simulink model "Pokus07_Display"  (Simulink 8.1)
settings: Solver=ode45  StartTime=0.0  StopTime=10.0  RelTol=1e-3
undefined symbols (not defined in the file): A, ARROW_DOWN, ARROW_LEFT, ARROW_RIGHT, ARROW_UP, ASTERISK, B, BACKSLASH, C, COLON, COMMA, CROSS, CURSOR, D, DOT, ending_column_index, ending_row_index, EQUAL, EXCLAMATION_MARK, F, framebuffer, G, GREATER_THAN, H, HEIGHT, hot, I, J, K, L, LEFT_PARENTHESES, LESS_THAN, M, MINUS, N, O, P, PERCENT, PLUS, POS_X, POS_Y, Q, QUESTION_MARK, QUOTE, R, RECTANGLE, RIGHT_PARENTHESES, S, SEMICOLON, SHARP, SLASH, SPACE, starting_column_index, starting_row_index, T, U, UNDERSCORE, V, W, WIDTH ... (+6)
libraries: dspmtrx3 x197, Common_Library x69, commutil2 x53, simulink_extras x1, dspsnks4 x1
(part 2 of 6)

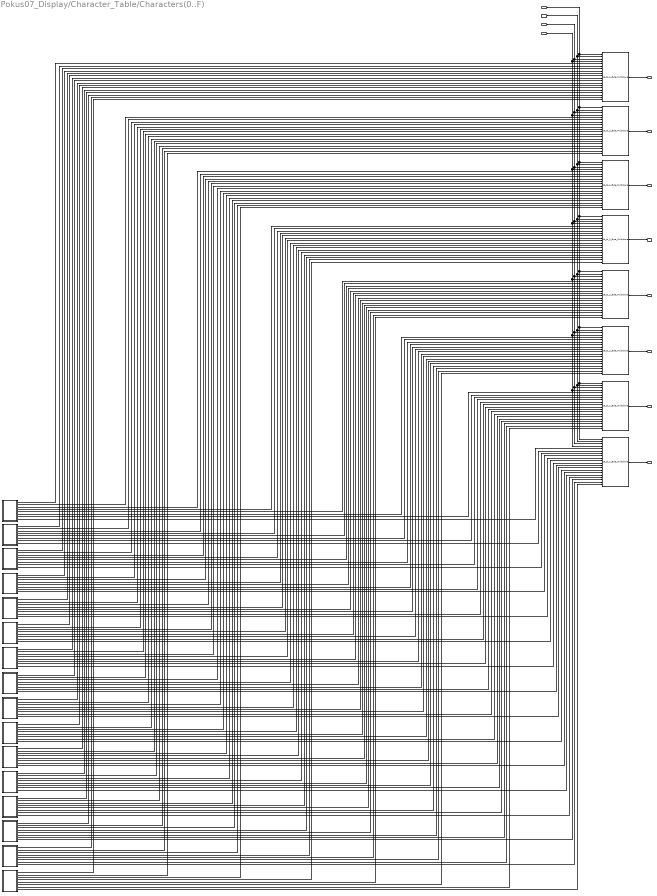
== system Pokus07_Display/Character_Table/Characters(0..F) ==
  Address_3_In(1b) : Inport
  Address_2_In(1b) : Inport  Port=2
  Address_1_In(1b) : Inport  Port=3
  Address_0_In(1b) : Inport  Port=4
  16_to_1_Byte_Multiplexer{,1..7} (8 alike) : Common_Library/Multiplexers/16_to_1_Byte_Multiplexer
  Char_0 : Subsystem
  Char_1 : Subsystem
  Char_2 : Subsystem
  Char_3 : Subsystem
  Char_4 : Subsystem
  Char_5 : Subsystem
  Char_6 : Subsystem
  Char_7 : Subsystem
  Char_8 : Subsystem
  Char_9 : Subsystem
  Char_A : Subsystem
  Char_B : Subsystem
  Char_C : Subsystem
  Char_D : Subsystem
  Char_E : Subsystem
  Char_F : Subsystem
  Column_1(1B) : Outport
  Column_2(1B) : Outport  Port=2
  Column_3(1B) : Outport  Port=3
  Column_4(1B) : Outport  Port=4
  Column_5(1B) : Outport  Port=5
  Column_6(1B) : Outport  Port=6
  Column_7(1B) : Outport  Port=7
  Column_8(1B) : Outport  Port=8
  wires:
  Char_F/1(Column_1(1B)) -> 16_to_1_Byte_Multiplexer/5
  Char_E/1(Column_1(1B)) -> 16_to_1_Byte_Multiplexer/6
  Char_D/1(Column_1(1B)) -> 16_to_1_Byte_Multiplexer/7
  Char_C/1(Column_1(1B)) -> 16_to_1_Byte_Multiplexer/8
  Char_B/1(Column_1(1B)) -> 16_to_1_Byte_Multiplexer/9
  Char_A/1(Column_1(1B)) -> 16_to_1_Byte_Multiplexer/10
  Char_9/1(Column_1(1B)) -> 16_to_1_Byte_Multiplexer/11
  Char_8/1(Column_1(1B)) -> 16_to_1_Byte_Multiplexer/12
  Char_7/1(Column_1(1B)) -> 16_to_1_Byte_Multiplexer/13
  Char_6/1(Column_1(1B)) -> 16_to_1_Byte_Multiplexer/14
  Char_5/1(Column_1(1B)) -> 16_to_1_Byte_Multiplexer/15
  Char_4/1(Column_1(1B)) -> 16_to_1_Byte_Multiplexer/16
  Char_3/1(Column_1(1B)) -> 16_to_1_Byte_Multiplexer/17
  Char_2/1(Column_1(1B)) -> 16_to_1_Byte_Multiplexer/18
  Char_1/1(Column_1(1B)) -> 16_to_1_Byte_Multiplexer/19
  Char_0/1(Column_1(1B)) -> 16_to_1_Byte_Multiplexer/20
  Char_F/2(Column_2(1B)) -> 16_to_1_Byte_Multiplexer1/5
  Char_0/2(Column_2(1B)) -> 16_to_1_Byte_Multiplexer1/20
  Char_1/2(Column_2(1B)) -> 16_to_1_Byte_Multiplexer1/19
  Char_2/2(Column_2(1B)) -> 16_to_1_Byte_Multiplexer1/18
  Char_3/2(Column_2(1B)) -> 16_to_1_Byte_Multiplexer1/17
  Char_4/2(Column_2(1B)) -> 16_to_1_Byte_Multiplexer1/16
  Char_5/2(Column_2(1B)) -> 16_to_1_Byte_Multiplexer1/15
  Char_6/2(Column_2(1B)) -> 16_to_1_Byte_Multiplexer1/14
  Char_7/2(Column_2(1B)) -> 16_to_1_Byte_Multiplexer1/13
  Char_8/2(Column_2(1B)) -> 16_to_1_Byte_Multiplexer1/12
  Char_9/2(Column_2(1B)) -> 16_to_1_Byte_Multiplexer1/11
  Char_A/2(Column_2(1B)) -> 16_to_1_Byte_Multiplexer1/10
  Char_B/2(Column_2(1B)) -> 16_to_1_Byte_Multiplexer1/9
  Char_C/2(Column_2(1B)) -> 16_to_1_Byte_Multiplexer1/8
  Char_D/2(Column_2(1B)) -> 16_to_1_Byte_Multiplexer1/7
  Char_E/2(Column_2(1B)) -> 16_to_1_Byte_Multiplexer1/6
  Char_0/3(Column_3(1B)) -> 16_to_1_Byte_Multiplexer2/20
  Char_1/3(Column_3(1B)) -> 16_to_1_Byte_Multiplexer2/19
  Char_2/3(Column_3(1B)) -> 16_to_1_Byte_Multiplexer2/18
  Char_3/3(Column_3(1B)) -> 16_to_1_Byte_Multiplexer2/17
  Char_4/3(Column_3(1B)) -> 16_to_1_Byte_Multiplexer2/16
  Char_5/3(Column_3(1B)) -> 16_to_1_Byte_Multiplexer2/15
  Char_6/3(Column_3(1B)) -> 16_to_1_Byte_Multiplexer2/14
  Char_7/3(Column_3(1B)) -> 16_to_1_Byte_Multiplexer2/13
  Char_8/3(Column_3(1B)) -> 16_to_1_Byte_Multiplexer2/12
  Char_9/3(Column_3(1B)) -> 16_to_1_Byte_Multiplexer2/11
  Char_A/3(Column_3(1B)) -> 16_to_1_Byte_Multiplexer2/10
  Char_B/3(Column_3(1B)) -> 16_to_1_Byte_Multiplexer2/9
  Char_C/3(Column_3(1B)) -> 16_to_1_Byte_Multiplexer2/8
  Char_D/3(Column_3(1B)) -> 16_to_1_Byte_Multiplexer2/7
  Char_E/3(Column_3(1B)) -> 16_to_1_Byte_Multiplexer2/6
  Char_F/3(Column_3(1B)) -> 16_to_1_Byte_Multiplexer2/5
  Char_0/4(Column_4(1B)) -> 16_to_1_Byte_Multiplexer3/20
  Char_1/4(Column_4(1B)) -> 16_to_1_Byte_Multiplexer3/19
  Char_2/4(Column_4(1B)) -> 16_to_1_Byte_Multiplexer3/18
  Char_3/4(Column_4(1B)) -> 16_to_1_Byte_Multiplexer3/17
  Char_4/4(Column_4(1B)) -> 16_to_1_Byte_Multiplexer3/16
  Char_5/4(Column_4(1B)) -> 16_to_1_Byte_Multiplexer3/15
  Char_6/4(Column_4(1B)) -> 16_to_1_Byte_Multiplexer3/14
  Char_7/4(Column_4(1B)) -> 16_to_1_Byte_Multiplexer3/13
  Char_8/4(Column_4(1B)) -> 16_to_1_Byte_Multiplexer3/12
  Char_9/4(Column_4(1B)) -> 16_to_1_Byte_Multiplexer3/11
  Char_A/4(Column_4(1B)) -> 16_to_1_Byte_Multiplexer3/10
  Char_B/4(Column_4(1B)) -> 16_to_1_Byte_Multiplexer3/9
  Char_C/4(Column_4(1B)) -> 16_to_1_Byte_Multiplexer3/8
  Char_D/4(Column_4(1B)) -> 16_to_1_Byte_Multiplexer3/7
  Char_E/4(Column_4(1B)) -> 16_to_1_Byte_Multiplexer3/6
  Char_F/4(Column_4(1B)) -> 16_to_1_Byte_Multiplexer3/5
  Char_0/5(Column_5(1B)) -> 16_to_1_Byte_Multiplexer4/20
  Char_1/5(Column_5(1B)) -> 16_to_1_Byte_Multiplexer4/19
  Char_2/5(Column_5(1B)) -> 16_to_1_Byte_Multiplexer4/18
  Char_3/5(Column_5(1B)) -> 16_to_1_Byte_Multiplexer4/17
  Char_4/5(Column_5(1B)) -> 16_to_1_Byte_Multiplexer4/16
  Char_5/5(Column_5(1B)) -> 16_to_1_Byte_Multiplexer4/15
  Char_7/5(Column_5(1B)) -> 16_to_1_Byte_Multiplexer4/13
  Char_6/5(Column_5(1B)) -> 16_to_1_Byte_Multiplexer4/14
  Char_8/5(Column_5(1B)) -> 16_to_1_Byte_Multiplexer4/12
  Char_9/5(Column_5(1B)) -> 16_to_1_Byte_Multiplexer4/11
  Char_A/5(Column_5(1B)) -> 16_to_1_Byte_Multiplexer4/10
  Char_B/5(Column_5(1B)) -> 16_to_1_Byte_Multiplexer4/9
  Char_C/5(Column_5(1B)) -> 16_to_1_Byte_Multiplexer4/8
  Char_D/5(Column_5(1B)) -> 16_to_1_Byte_Multiplexer4/7
  Char_E/5(Column_5(1B)) -> 16_to_1_Byte_Multiplexer4/6
  Char_F/5(Column_5(1B)) -> 16_to_1_Byte_Multiplexer4/5
  Char_0/6(Column_6(1B)) -> 16_to_1_Byte_Multiplexer5/20
  Char_1/6(Column_6(1B)) -> 16_to_1_Byte_Multiplexer5/19
  Char_2/6(Column_6(1B)) -> 16_to_1_Byte_Multiplexer5/18
  Char_3/6(Column_6(1B)) -> 16_to_1_Byte_Multiplexer5/17
  Char_4/6(Column_6(1B)) -> 16_to_1_Byte_Multiplexer5/16
  Char_5/6(Column_6(1B)) -> 16_to_1_Byte_Multiplexer5/15
  Char_6/6(Column_6(1B)) -> 16_to_1_Byte_Multiplexer5/14
  Char_7/6(Column_6(1B)) -> 16_to_1_Byte_Multiplexer5/13
  Char_8/6(Column_6(1B)) -> 16_to_1_Byte_Multiplexer5/12
  Char_9/6(Column_6(1B)) -> 16_to_1_Byte_Multiplexer5/11
  Char_A/6(Column_6(1B)) -> 16_to_1_Byte_Multiplexer5/10
  Char_B/6(Column_6(1B)) -> 16_to_1_Byte_Multiplexer5/9
  Char_C/7(Column_7(1B)) -> 16_to_1_Byte_Multiplexer6/8
  Char_C/6(Column_6(1B)) -> 16_to_1_Byte_Multiplexer5/8
  Char_D/6(Column_6(1B)) -> 16_to_1_Byte_Multiplexer5/7
  Char_E/6(Column_6(1B)) -> 16_to_1_Byte_Multiplexer5/6
  Char_F/6(Column_6(1B)) -> 16_to_1_Byte_Multiplexer5/5
  Char_0/7(Column_7(1B)) -> 16_to_1_Byte_Multiplexer6/20
  Char_1/7(Column_7(1B)) -> 16_to_1_Byte_Multiplexer6/19
  Char_2/7(Column_7(1B)) -> 16_to_1_Byte_Multiplexer6/18
  Char_3/7(Column_7(1B)) -> 16_to_1_Byte_Multiplexer6/17
  Char_4/7(Column_7(1B)) -> 16_to_1_Byte_Multiplexer6/16
  Char_5/7(Column_7(1B)) -> 16_to_1_Byte_Multiplexer6/15
  Char_6/7(Column_7(1B)) -> 16_to_1_Byte_Multiplexer6/14
  Char_7/7(Column_7(1B)) -> 16_to_1_Byte_Multiplexer6/13
  Char_8/7(Column_7(1B)) -> 16_to_1_Byte_Multiplexer6/12
  Char_9/7(Column_7(1B)) -> 16_to_1_Byte_Multiplexer6/11
  Char_A/7(Column_7(1B)) -> 16_to_1_Byte_Multiplexer6/10
  Char_B/7(Column_7(1B)) -> 16_to_1_Byte_Multiplexer6/9
  Char_D/7(Column_7(1B)) -> 16_to_1_Byte_Multiplexer6/7
  Char_E/7(Column_7(1B)) -> 16_to_1_Byte_Multiplexer6/6
  Char_F/7(Column_7(1B)) -> 16_to_1_Byte_Multiplexer6/5
  Char_0/8(Column_8(1B)) -> 16_to_1_Byte_Multiplexer7/20
  Char_1/8(Column_8(1B)) -> 16_to_1_Byte_Multiplexer7/19
  Char_2/8(Column_8(1B)) -> 16_to_1_Byte_Multiplexer7/18
  Char_3/8(Column_8(1B)) -> 16_to_1_Byte_Multiplexer7/17
  Char_4/8(Column_8(1B)) -> 16_to_1_Byte_Multiplexer7/16
  Char_5/8(Column_8(1B)) -> 16_to_1_Byte_Multiplexer7/15
  Char_6/8(Column_8(1B)) -> 16_to_1_Byte_Multiplexer7/14
  Char_7/8(Column_8(1B)) -> 16_to_1_Byte_Multiplexer7/13
  Char_8/8(Column_8(1B)) -> 16_to_1_Byte_Multiplexer7/12
  Char_9/8(Column_8(1B)) -> 16_to_1_Byte_Multiplexer7/11
  Char_A/8(Column_8(1B)) -> 16_to_1_Byte_Multiplexer7/10
  Char_B/8(Column_8(1B)) -> 16_to_1_Byte_Multiplexer7/9
  Char_C/8(Column_8(1B)) -> 16_to_1_Byte_Multiplexer7/8
  Char_D/8(Column_8(1B)) -> 16_to_1_Byte_Multiplexer7/7
  Char_E/8(Column_8(1B)) -> 16_to_1_Byte_Multiplexer7/6
  Char_F/8(Column_8(1B)) -> 16_to_1_Byte_Multiplexer7/5
  16_to_1_Byte_Multiplexer/1 -> Column_1(1B)/1
  16_to_1_Byte_Multiplexer1/1 -> Column_2(1B)/1
  16_to_1_Byte_Multiplexer2/1 -> Column_3(1B)/1
  16_to_1_Byte_Multiplexer3/1 -> Column_4(1B)/1
  16_to_1_Byte_Multiplexer4/1 -> Column_5(1B)/1
  16_to_1_Byte_Multiplexer5/1 -> Column_6(1B)/1
  16_to_1_Byte_Multiplexer6/1 -> Column_7(1B)/1
  16_to_1_Byte_Multiplexer7/1 -> Column_8(1B)/1
  Address_0_In(1b)/1 -> 16_to_1_Byte_Multiplexer/4, 16_to_1_Byte_Multiplexer1/4, 16_to_1_Byte_Multiplexer2/4, 16_to_1_Byte_Multiplexer3/4, 16_to_1_Byte_Multiplexer4/4, 16_to_1_Byte_Multiplexer5/4, 16_to_1_Byte_Multiplexer6/4, 16_to_1_Byte_Multiplexer7/4
  Address_1_In(1b)/1 -> 16_to_1_Byte_Multiplexer/3, 16_to_1_Byte_Multiplexer1/3, 16_to_1_Byte_Multiplexer2/3, 16_to_1_Byte_Multiplexer3/3, 16_to_1_Byte_Multiplexer4/3, 16_to_1_Byte_Multiplexer5/3, 16_to_1_Byte_Multiplexer6/3, 16_to_1_Byte_Multiplexer7/3
  Address_2_In(1b)/1 -> 16_to_1_Byte_Multiplexer/2, 16_to_1_Byte_Multiplexer1/2, 16_to_1_Byte_Multiplexer2/2, 16_to_1_Byte_Multiplexer3/2, 16_to_1_Byte_Multiplexer4/2, 16_to_1_Byte_Multiplexer5/2, 16_to_1_Byte_Multiplexer6/2, 16_to_1_Byte_Multiplexer7/2
  Address_3_In(1b)/1 -> 16_to_1_Byte_Multiplexer/1, 16_to_1_Byte_Multiplexer1/1, 16_to_1_Byte_Multiplexer2/1, 16_to_1_Byte_Multiplexer3/1, 16_to_1_Byte_Multiplexer4/1, 16_to_1_Byte_Multiplexer5/1, 16_to_1_Byte_Multiplexer6/1, 16_to_1_Byte_Multiplexer7/1

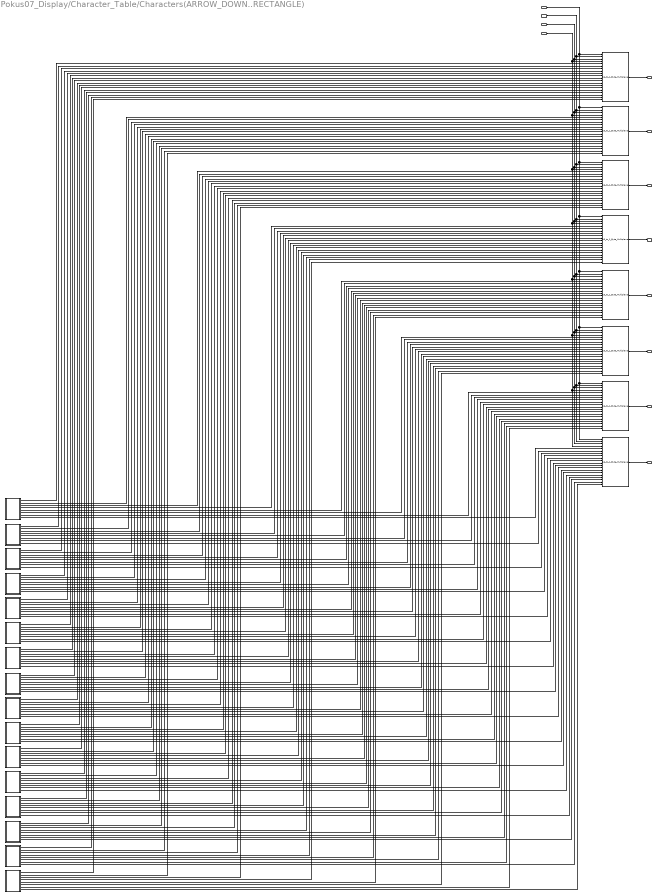
== system Pokus07_Display/Character_Table/Characters(ARROW_DOWN..RECTANGLE) ==
  Address_3_In(1b) : Inport
  Address_2_In(1b) : Inport  Port=2
  Address_1_In(1b) : Inport  Port=3
  Address_0_In(1b) : Inport  Port=4
  16_to_1_Byte_Multiplexer{,1..7} (8 alike) : Common_Library/Multiplexers/16_to_1_Byte_Multiplexer
  Char_ARROW_DOWN : Subsystem
  Char_ARROW_LEFT : Subsystem
  Char_ARROW_RIGHT : Subsystem
  Char_COMMA : Subsystem
  Char_CURSOR : Subsystem
  Char_DOT : Subsystem
  Char_EXCLAMATION_MARK : Subsystem
  Char_LEFT_PARENTHESES : Subsystem
  Char_PERCENT : Subsystem
  Char_QUESTION_MARK : Subsystem
  Char_QUOTE : Subsystem
  Char_RECTANGLE : Subsystem
  Char_RIGHT_PARENTHESES : Subsystem
  Char_SHARP : Subsystem
  Char_SPACE : Subsystem
  Char_UNDERSCORE : Subsystem
  Column_1(1B) : Outport
  Column_2(1B) : Outport  Port=2
  Column_3(1B) : Outport  Port=3
  Column_4(1B) : Outport  Port=4
  Column_5(1B) : Outport  Port=5
  Column_6(1B) : Outport  Port=6
  Column_7(1B) : Outport  Port=7
  Column_8(1B) : Outport  Port=8
  wires:
  Char_RECTANGLE/1(Column_1(1B)) -> 16_to_1_Byte_Multiplexer/5
  Char_CURSOR/1(Column_1(1B)) -> 16_to_1_Byte_Multiplexer/6
  Char_SPACE/1(Column_1(1B)) -> 16_to_1_Byte_Multiplexer/7
  Char_RIGHT_PARENTHESES/1(Column_1(1B)) -> 16_to_1_Byte_Multiplexer/8
  Char_LEFT_PARENTHESES/1(Column_1(1B)) -> 16_to_1_Byte_Multiplexer/9
  Char_PERCENT/1(Column_1(1B)) -> 16_to_1_Byte_Multiplexer/10
  Char_SHARP/1(Column_1(1B)) -> 16_to_1_Byte_Multiplexer/11
  Char_QUOTE/1(Column_1(1B)) -> 16_to_1_Byte_Multiplexer/12
  Char_EXCLAMATION_MARK/1(Column_1(1B)) -> 16_to_1_Byte_Multiplexer/13
  Char_QUESTION_MARK/1(Column_1(1B)) -> 16_to_1_Byte_Multiplexer/14
  Char_COMMA/1(Column_1(1B)) -> 16_to_1_Byte_Multiplexer/15
  Char_DOT/1(Column_1(1B)) -> 16_to_1_Byte_Multiplexer/16
  Char_UNDERSCORE/1(Column_1(1B)) -> 16_to_1_Byte_Multiplexer/17
  Char_ARROW_RIGHT/1(Column_1(1B)) -> 16_to_1_Byte_Multiplexer/18
  Char_ARROW_LEFT/1(Column_1(1B)) -> 16_to_1_Byte_Multiplexer/19
  Char_ARROW_DOWN/1(Column_1(1B)) -> 16_to_1_Byte_Multiplexer/20
  Char_RECTANGLE/2(Column_2(1B)) -> 16_to_1_Byte_Multiplexer1/5
  Char_ARROW_DOWN/2(Column_2(1B)) -> 16_to_1_Byte_Multiplexer1/20
  Char_ARROW_LEFT/2(Column_2(1B)) -> 16_to_1_Byte_Multiplexer1/19
  Char_ARROW_RIGHT/2(Column_2(1B)) -> 16_to_1_Byte_Multiplexer1/18
  Char_UNDERSCORE/2(Column_2(1B)) -> 16_to_1_Byte_Multiplexer1/17
  Char_DOT/2(Column_2(1B)) -> 16_to_1_Byte_Multiplexer1/16
  Char_COMMA/2(Column_2(1B)) -> 16_to_1_Byte_Multiplexer1/15
  Char_QUESTION_MARK/2(Column_2(1B)) -> 16_to_1_Byte_Multiplexer1/14
  Char_EXCLAMATION_MARK/2(Column_2(1B)) -> 16_to_1_Byte_Multiplexer1/13
  Char_QUOTE/2(Column_2(1B)) -> 16_to_1_Byte_Multiplexer1/12
  Char_SHARP/2(Column_2(1B)) -> 16_to_1_Byte_Multiplexer1/11
  Char_PERCENT/2(Column_2(1B)) -> 16_to_1_Byte_Multiplexer1/10
  Char_LEFT_PARENTHESES/2(Column_2(1B)) -> 16_to_1_Byte_Multiplexer1/9
  Char_RIGHT_PARENTHESES/2(Column_2(1B)) -> 16_to_1_Byte_Multiplexer1/8
  Char_SPACE/2(Column_2(1B)) -> 16_to_1_Byte_Multiplexer1/7
  Char_CURSOR/2(Column_2(1B)) -> 16_to_1_Byte_Multiplexer1/6
  Char_ARROW_DOWN/3(Column_3(1B)) -> 16_to_1_Byte_Multiplexer2/20
  Char_ARROW_LEFT/3(Column_3(1B)) -> 16_to_1_Byte_Multiplexer2/19
  Char_ARROW_RIGHT/3(Column_3(1B)) -> 16_to_1_Byte_Multiplexer2/18
  Char_UNDERSCORE/3(Column_3(1B)) -> 16_to_1_Byte_Multiplexer2/17
  Char_DOT/3(Column_3(1B)) -> 16_to_1_Byte_Multiplexer2/16
  Char_COMMA/3(Column_3(1B)) -> 16_to_1_Byte_Multiplexer2/15
  Char_QUESTION_MARK/3(Column_3(1B)) -> 16_to_1_Byte_Multiplexer2/14
  Char_EXCLAMATION_MARK/3(Column_3(1B)) -> 16_to_1_Byte_Multiplexer2/13
  Char_QUOTE/3(Column_3(1B)) -> 16_to_1_Byte_Multiplexer2/12
  Char_SHARP/3(Column_3(1B)) -> 16_to_1_Byte_Multiplexer2/11
  Char_PERCENT/3(Column_3(1B)) -> 16_to_1_Byte_Multiplexer2/10
  Char_LEFT_PARENTHESES/3(Column_3(1B)) -> 16_to_1_Byte_Multiplexer2/9
  Char_RIGHT_PARENTHESES/3(Column_3(1B)) -> 16_to_1_Byte_Multiplexer2/8
  Char_SPACE/3(Column_3(1B)) -> 16_to_1_Byte_Multiplexer2/7
  Char_CURSOR/3(Column_3(1B)) -> 16_to_1_Byte_Multiplexer2/6
  Char_RECTANGLE/3(Column_3(1B)) -> 16_to_1_Byte_Multiplexer2/5
  Char_ARROW_DOWN/4(Column_4(1B)) -> 16_to_1_Byte_Multiplexer3/20
  Char_ARROW_LEFT/4(Column_4(1B)) -> 16_to_1_Byte_Multiplexer3/19
  Char_ARROW_RIGHT/4(Column_4(1B)) -> 16_to_1_Byte_Multiplexer3/18
  Char_UNDERSCORE/4(Column_4(1B)) -> 16_to_1_Byte_Multiplexer3/17
  Char_DOT/4(Column_4(1B)) -> 16_to_1_Byte_Multiplexer3/16
  Char_COMMA/4(Column_4(1B)) -> 16_to_1_Byte_Multiplexer3/15
  Char_QUESTION_MARK/4(Column_4(1B)) -> 16_to_1_Byte_Multiplexer3/14
  Char_EXCLAMATION_MARK/4(Column_4(1B)) -> 16_to_1_Byte_Multiplexer3/13
  Char_QUOTE/4(Column_4(1B)) -> 16_to_1_Byte_Multiplexer3/12
  Char_SHARP/4(Column_4(1B)) -> 16_to_1_Byte_Multiplexer3/11
  Char_PERCENT/4(Column_4(1B)) -> 16_to_1_Byte_Multiplexer3/10
  Char_LEFT_PARENTHESES/4(Column_4(1B)) -> 16_to_1_Byte_Multiplexer3/9
  Char_RIGHT_PARENTHESES/4(Column_4(1B)) -> 16_to_1_Byte_Multiplexer3/8
  Char_SPACE/4(Column_4(1B)) -> 16_to_1_Byte_Multiplexer3/7
  Char_CURSOR/4(Column_4(1B)) -> 16_to_1_Byte_Multiplexer3/6
  Char_RECTANGLE/4(Column_4(1B)) -> 16_to_1_Byte_Multiplexer3/5
  Char_ARROW_DOWN/5(Column_5(1B)) -> 16_to_1_Byte_Multiplexer4/20
  Char_ARROW_LEFT/5(Column_5(1B)) -> 16_to_1_Byte_Multiplexer4/19
  Char_ARROW_RIGHT/5(Column_5(1B)) -> 16_to_1_Byte_Multiplexer4/18
  Char_UNDERSCORE/5(Column_5(1B)) -> 16_to_1_Byte_Multiplexer4/17
  Char_DOT/5(Column_5(1B)) -> 16_to_1_Byte_Multiplexer4/16
  Char_COMMA/5(Column_5(1B)) -> 16_to_1_Byte_Multiplexer4/15
  Char_EXCLAMATION_MARK/5(Column_5(1B)) -> 16_to_1_Byte_Multiplexer4/13
  Char_QUESTION_MARK/5(Column_5(1B)) -> 16_to_1_Byte_Multiplexer4/14
  Char_QUOTE/5(Column_5(1B)) -> 16_to_1_Byte_Multiplexer4/12
  Char_SHARP/5(Column_5(1B)) -> 16_to_1_Byte_Multiplexer4/11
  Char_PERCENT/5(Column_5(1B)) -> 16_to_1_Byte_Multiplexer4/10
  Char_LEFT_PARENTHESES/5(Column_5(1B)) -> 16_to_1_Byte_Multiplexer4/9
  Char_RIGHT_PARENTHESES/5(Column_5(1B)) -> 16_to_1_Byte_Multiplexer4/8
  Char_SPACE/5(Column_5(1B)) -> 16_to_1_Byte_Multiplexer4/7
  Char_CURSOR/5(Column_5(1B)) -> 16_to_1_Byte_Multiplexer4/6
  Char_RECTANGLE/5(Column_5(1B)) -> 16_to_1_Byte_Multiplexer4/5
  Char_ARROW_DOWN/6(Column_6(1B)) -> 16_to_1_Byte_Multiplexer5/20
  Char_ARROW_LEFT/6(Column_6(1B)) -> 16_to_1_Byte_Multiplexer5/19
  Char_ARROW_RIGHT/6(Column_6(1B)) -> 16_to_1_Byte_Multiplexer5/18
  Char_UNDERSCORE/6(Column_6(1B)) -> 16_to_1_Byte_Multiplexer5/17
  Char_DOT/6(Column_6(1B)) -> 16_to_1_Byte_Multiplexer5/16
  Char_COMMA/6(Column_6(1B)) -> 16_to_1_Byte_Multiplexer5/15
  Char_QUESTION_MARK/6(Column_6(1B)) -> 16_to_1_Byte_Multiplexer5/14
  Char_EXCLAMATION_MARK/6(Column_6(1B)) -> 16_to_1_Byte_Multiplexer5/13
  Char_QUOTE/6(Column_6(1B)) -> 16_to_1_Byte_Multiplexer5/12
  Char_SHARP/6(Column_6(1B)) -> 16_to_1_Byte_Multiplexer5/11
  Char_PERCENT/6(Column_6(1B)) -> 16_to_1_Byte_Multiplexer5/10
  Char_LEFT_PARENTHESES/6(Column_6(1B)) -> 16_to_1_Byte_Multiplexer5/9
  Char_RIGHT_PARENTHESES/7(Column_7(1B)) -> 16_to_1_Byte_Multiplexer6/8
  Char_RIGHT_PARENTHESES/6(Column_6(1B)) -> 16_to_1_Byte_Multiplexer5/8
  Char_SPACE/6(Column_6(1B)) -> 16_to_1_Byte_Multiplexer5/7
  Char_CURSOR/6(Column_6(1B)) -> 16_to_1_Byte_Multiplexer5/6
  Char_RECTANGLE/6(Column_6(1B)) -> 16_to_1_Byte_Multiplexer5/5
  Char_ARROW_DOWN/7(Column_7(1B)) -> 16_to_1_Byte_Multiplexer6/20
  Char_ARROW_LEFT/7(Column_7(1B)) -> 16_to_1_Byte_Multiplexer6/19
  Char_ARROW_RIGHT/7(Column_7(1B)) -> 16_to_1_Byte_Multiplexer6/18
  Char_UNDERSCORE/7(Column_7(1B)) -> 16_to_1_Byte_Multiplexer6/17
  Char_DOT/7(Column_7(1B)) -> 16_to_1_Byte_Multiplexer6/16
  Char_COMMA/7(Column_7(1B)) -> 16_to_1_Byte_Multiplexer6/15
  Char_QUESTION_MARK/7(Column_7(1B)) -> 16_to_1_Byte_Multiplexer6/14
  Char_EXCLAMATION_MARK/7(Column_7(1B)) -> 16_to_1_Byte_Multiplexer6/13
  Char_QUOTE/7(Column_7(1B)) -> 16_to_1_Byte_Multiplexer6/12
  Char_SHARP/7(Column_7(1B)) -> 16_to_1_Byte_Multiplexer6/11
  Char_PERCENT/7(Column_7(1B)) -> 16_to_1_Byte_Multiplexer6/10
  Char_LEFT_PARENTHESES/7(Column_7(1B)) -> 16_to_1_Byte_Multiplexer6/9
  Char_SPACE/7(Column_7(1B)) -> 16_to_1_Byte_Multiplexer6/7
  Char_CURSOR/7(Column_7(1B)) -> 16_to_1_Byte_Multiplexer6/6
  Char_RECTANGLE/7(Column_7(1B)) -> 16_to_1_Byte_Multiplexer6/5
  Char_ARROW_DOWN/8(Column_8(1B)) -> 16_to_1_Byte_Multiplexer7/20
  Char_ARROW_LEFT/8(Column_8(1B)) -> 16_to_1_Byte_Multiplexer7/19
  Char_ARROW_RIGHT/8(Column_8(1B)) -> 16_to_1_Byte_Multiplexer7/18
  Char_UNDERSCORE/8(Column_8(1B)) -> 16_to_1_Byte_Multiplexer7/17
  Char_DOT/8(Column_8(1B)) -> 16_to_1_Byte_Multiplexer7/16
  Char_COMMA/8(Column_8(1B)) -> 16_to_1_Byte_Multiplexer7/15
  Char_QUESTION_MARK/8(Column_8(1B)) -> 16_to_1_Byte_Multiplexer7/14
  Char_EXCLAMATION_MARK/8(Column_8(1B)) -> 16_to_1_Byte_Multiplexer7/13
  Char_QUOTE/8(Column_8(1B)) -> 16_to_1_Byte_Multiplexer7/12
  Char_SHARP/8(Column_8(1B)) -> 16_to_1_Byte_Multiplexer7/11
  Char_PERCENT/8(Column_8(1B)) -> 16_to_1_Byte_Multiplexer7/10
  Char_LEFT_PARENTHESES/8(Column_8(1B)) -> 16_to_1_Byte_Multiplexer7/9
  Char_RIGHT_PARENTHESES/8(Column_8(1B)) -> 16_to_1_Byte_Multiplexer7/8
  Char_SPACE/8(Column_8(1B)) -> 16_to_1_Byte_Multiplexer7/7
  Char_CURSOR/8(Column_8(1B)) -> 16_to_1_Byte_Multiplexer7/6
  Char_RECTANGLE/8(Column_8(1B)) -> 16_to_1_Byte_Multiplexer7/5
  16_to_1_Byte_Multiplexer/1 -> Column_1(1B)/1
  16_to_1_Byte_Multiplexer1/1 -> Column_2(1B)/1
  16_to_1_Byte_Multiplexer2/1 -> Column_3(1B)/1
  16_to_1_Byte_Multiplexer3/1 -> Column_4(1B)/1
  16_to_1_Byte_Multiplexer4/1 -> Column_5(1B)/1
  16_to_1_Byte_Multiplexer5/1 -> Column_6(1B)/1
  16_to_1_Byte_Multiplexer6/1 -> Column_7(1B)/1
  16_to_1_Byte_Multiplexer7/1 -> Column_8(1B)/1
  Address_0_In(1b)/1 -> 16_to_1_Byte_Multiplexer/4, 16_to_1_Byte_Multiplexer1/4, 16_to_1_Byte_Multiplexer2/4, 16_to_1_Byte_Multiplexer3/4, 16_to_1_Byte_Multiplexer4/4, 16_to_1_Byte_Multiplexer5/4, 16_to_1_Byte_Multiplexer6/4, 16_to_1_Byte_Multiplexer7/4
  Address_1_In(1b)/1 -> 16_to_1_Byte_Multiplexer/3, 16_to_1_Byte_Multiplexer1/3, 16_to_1_Byte_Multiplexer2/3, 16_to_1_Byte_Multiplexer3/3, 16_to_1_Byte_Multiplexer4/3, 16_to_1_Byte_Multiplexer5/3, 16_to_1_Byte_Multiplexer6/3, 16_to_1_Byte_Multiplexer7/3
  Address_2_In(1b)/1 -> 16_to_1_Byte_Multiplexer/2, 16_to_1_Byte_Multiplexer1/2, 16_to_1_Byte_Multiplexer2/2, 16_to_1_Byte_Multiplexer3/2, 16_to_1_Byte_Multiplexer4/2, 16_to_1_Byte_Multiplexer5/2, 16_to_1_Byte_Multiplexer6/2, 16_to_1_Byte_Multiplexer7/2
  Address_3_In(1b)/1 -> 16_to_1_Byte_Multiplexer/1, 16_to_1_Byte_Multiplexer1/1, 16_to_1_Byte_Multiplexer2/1, 16_to_1_Byte_Multiplexer3/1, 16_to_1_Byte_Multiplexer4/1, 16_to_1_Byte_Multiplexer5/1, 16_to_1_Byte_Multiplexer6/1, 16_to_1_Byte_Multiplexer7/1

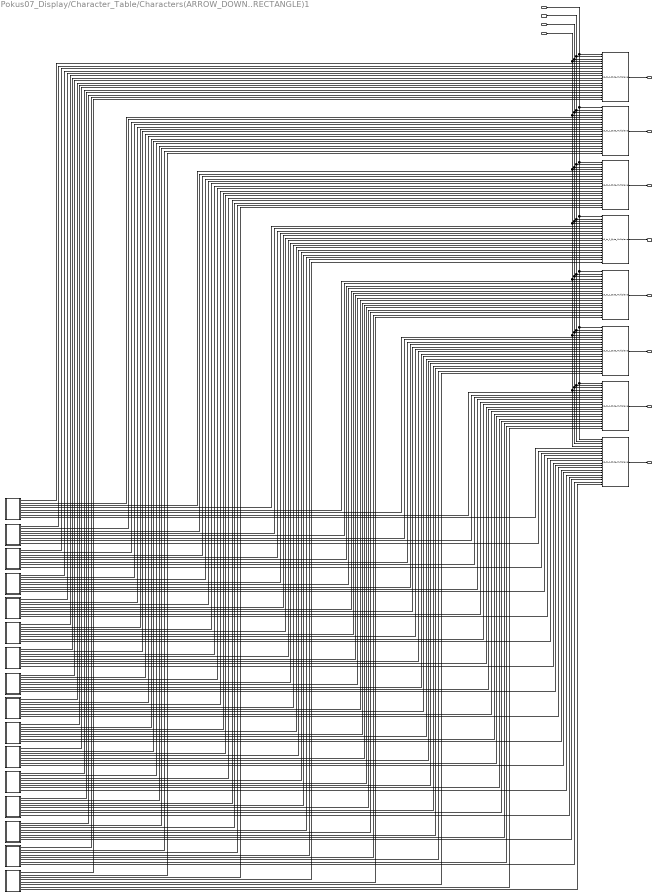
== system Pokus07_Display/Character_Table/Characters(ARROW_DOWN..RECTANGLE)1 ==
  Address_3_In(1b) : Inport
  Address_2_In(1b) : Inport  Port=2
  Address_1_In(1b) : Inport  Port=3
  Address_0_In(1b) : Inport  Port=4
  16_to_1_Byte_Multiplexer{,1..7} (8 alike) : Common_Library/Multiplexers/16_to_1_Byte_Multiplexer
  Char_ARROW_DOWN : Subsystem
  Char_ARROW_LEFT : Subsystem
  Char_ARROW_RIGHT : Subsystem
  Char_COMMA : Subsystem
  Char_CURSOR : Subsystem
  Char_DOT : Subsystem
  Char_EXCLAMATION_MARK : Subsystem
  Char_LEFT_PARENTHESES : Subsystem
  Char_PERCENT : Subsystem
  Char_QUESTION_MARK : Subsystem
  Char_QUOTE : Subsystem
  Char_RECTANGLE : Subsystem
  Char_RIGHT_PARENTHESES : Subsystem
  Char_SHARP : Subsystem
  Char_SPACE : Subsystem
  Char_UNDERSCORE : Subsystem
  Column_1(1B) : Outport
  Column_2(1B) : Outport  Port=2
  Column_3(1B) : Outport  Port=3
  Column_4(1B) : Outport  Port=4
  Column_5(1B) : Outport  Port=5
  Column_6(1B) : Outport  Port=6
  Column_7(1B) : Outport  Port=7
  Column_8(1B) : Outport  Port=8
  wires:
  Char_RECTANGLE/1(Column_1(1B)) -> 16_to_1_Byte_Multiplexer/5
  Char_CURSOR/1(Column_1(1B)) -> 16_to_1_Byte_Multiplexer/6
  Char_SPACE/1(Column_1(1B)) -> 16_to_1_Byte_Multiplexer/7
  Char_RIGHT_PARENTHESES/1(Column_1(1B)) -> 16_to_1_Byte_Multiplexer/8
  Char_LEFT_PARENTHESES/1(Column_1(1B)) -> 16_to_1_Byte_Multiplexer/9
  Char_PERCENT/1(Column_1(1B)) -> 16_to_1_Byte_Multiplexer/10
  Char_SHARP/1(Column_1(1B)) -> 16_to_1_Byte_Multiplexer/11
  Char_QUOTE/1(Column_1(1B)) -> 16_to_1_Byte_Multiplexer/12
  Char_EXCLAMATION_MARK/1(Column_1(1B)) -> 16_to_1_Byte_Multiplexer/13
  Char_QUESTION_MARK/1(Column_1(1B)) -> 16_to_1_Byte_Multiplexer/14
  Char_COMMA/1(Column_1(1B)) -> 16_to_1_Byte_Multiplexer/15
  Char_DOT/1(Column_1(1B)) -> 16_to_1_Byte_Multiplexer/16
  Char_UNDERSCORE/1(Column_1(1B)) -> 16_to_1_Byte_Multiplexer/17
  Char_ARROW_RIGHT/1(Column_1(1B)) -> 16_to_1_Byte_Multiplexer/18
  Char_ARROW_LEFT/1(Column_1(1B)) -> 16_to_1_Byte_Multiplexer/19
  Char_ARROW_DOWN/1(Column_1(1B)) -> 16_to_1_Byte_Multiplexer/20
  Char_RECTANGLE/2(Column_2(1B)) -> 16_to_1_Byte_Multiplexer1/5
  Char_ARROW_DOWN/2(Column_2(1B)) -> 16_to_1_Byte_Multiplexer1/20
  Char_ARROW_LEFT/2(Column_2(1B)) -> 16_to_1_Byte_Multiplexer1/19
  Char_ARROW_RIGHT/2(Column_2(1B)) -> 16_to_1_Byte_Multiplexer1/18
  Char_UNDERSCORE/2(Column_2(1B)) -> 16_to_1_Byte_Multiplexer1/17
  Char_DOT/2(Column_2(1B)) -> 16_to_1_Byte_Multiplexer1/16
  Char_COMMA/2(Column_2(1B)) -> 16_to_1_Byte_Multiplexer1/15
  Char_QUESTION_MARK/2(Column_2(1B)) -> 16_to_1_Byte_Multiplexer1/14
  Char_EXCLAMATION_MARK/2(Column_2(1B)) -> 16_to_1_Byte_Multiplexer1/13
  Char_QUOTE/2(Column_2(1B)) -> 16_to_1_Byte_Multiplexer1/12
  Char_SHARP/2(Column_2(1B)) -> 16_to_1_Byte_Multiplexer1/11
  Char_PERCENT/2(Column_2(1B)) -> 16_to_1_Byte_Multiplexer1/10
  Char_LEFT_PARENTHESES/2(Column_2(1B)) -> 16_to_1_Byte_Multiplexer1/9
  Char_RIGHT_PARENTHESES/2(Column_2(1B)) -> 16_to_1_Byte_Multiplexer1/8
  Char_SPACE/2(Column_2(1B)) -> 16_to_1_Byte_Multiplexer1/7
  Char_CURSOR/2(Column_2(1B)) -> 16_to_1_Byte_Multiplexer1/6
  Char_ARROW_DOWN/3(Column_3(1B)) -> 16_to_1_Byte_Multiplexer2/20
  Char_ARROW_LEFT/3(Column_3(1B)) -> 16_to_1_Byte_Multiplexer2/19
  Char_ARROW_RIGHT/3(Column_3(1B)) -> 16_to_1_Byte_Multiplexer2/18
  Char_UNDERSCORE/3(Column_3(1B)) -> 16_to_1_Byte_Multiplexer2/17
  Char_DOT/3(Column_3(1B)) -> 16_to_1_Byte_Multiplexer2/16
  Char_COMMA/3(Column_3(1B)) -> 16_to_1_Byte_Multiplexer2/15
  Char_QUESTION_MARK/3(Column_3(1B)) -> 16_to_1_Byte_Multiplexer2/14
  Char_EXCLAMATION_MARK/3(Column_3(1B)) -> 16_to_1_Byte_Multiplexer2/13
  Char_QUOTE/3(Column_3(1B)) -> 16_to_1_Byte_Multiplexer2/12
  Char_SHARP/3(Column_3(1B)) -> 16_to_1_Byte_Multiplexer2/11
  Char_PERCENT/3(Column_3(1B)) -> 16_to_1_Byte_Multiplexer2/10
  Char_LEFT_PARENTHESES/3(Column_3(1B)) -> 16_to_1_Byte_Multiplexer2/9
  Char_RIGHT_PARENTHESES/3(Column_3(1B)) -> 16_to_1_Byte_Multiplexer2/8
  Char_SPACE/3(Column_3(1B)) -> 16_to_1_Byte_Multiplexer2/7
  Char_CURSOR/3(Column_3(1B)) -> 16_to_1_Byte_Multiplexer2/6
  Char_RECTANGLE/3(Column_3(1B)) -> 16_to_1_Byte_Multiplexer2/5
  Char_ARROW_DOWN/4(Column_4(1B)) -> 16_to_1_Byte_Multiplexer3/20
  Char_ARROW_LEFT/4(Column_4(1B)) -> 16_to_1_Byte_Multiplexer3/19
  Char_ARROW_RIGHT/4(Column_4(1B)) -> 16_to_1_Byte_Multiplexer3/18
  Char_UNDERSCORE/4(Column_4(1B)) -> 16_to_1_Byte_Multiplexer3/17
  Char_DOT/4(Column_4(1B)) -> 16_to_1_Byte_Multiplexer3/16
  Char_COMMA/4(Column_4(1B)) -> 16_to_1_Byte_Multiplexer3/15
  Char_QUESTION_MARK/4(Column_4(1B)) -> 16_to_1_Byte_Multiplexer3/14
  Char_EXCLAMATION_MARK/4(Column_4(1B)) -> 16_to_1_Byte_Multiplexer3/13
  Char_QUOTE/4(Column_4(1B)) -> 16_to_1_Byte_Multiplexer3/12
  Char_SHARP/4(Column_4(1B)) -> 16_to_1_Byte_Multiplexer3/11
  Char_PERCENT/4(Column_4(1B)) -> 16_to_1_Byte_Multiplexer3/10
  Char_LEFT_PARENTHESES/4(Column_4(1B)) -> 16_to_1_Byte_Multiplexer3/9
  Char_RIGHT_PARENTHESES/4(Column_4(1B)) -> 16_to_1_Byte_Multiplexer3/8
  Char_SPACE/4(Column_4(1B)) -> 16_to_1_Byte_Multiplexer3/7
  Char_CURSOR/4(Column_4(1B)) -> 16_to_1_Byte_Multiplexer3/6
  Char_RECTANGLE/4(Column_4(1B)) -> 16_to_1_Byte_Multiplexer3/5
  Char_ARROW_DOWN/5(Column_5(1B)) -> 16_to_1_Byte_Multiplexer4/20
  Char_ARROW_LEFT/5(Column_5(1B)) -> 16_to_1_Byte_Multiplexer4/19
  Char_ARROW_RIGHT/5(Column_5(1B)) -> 16_to_1_Byte_Multiplexer4/18
  Char_UNDERSCORE/5(Column_5(1B)) -> 16_to_1_Byte_Multiplexer4/17
  Char_DOT/5(Column_5(1B)) -> 16_to_1_Byte_Multiplexer4/16
  Char_COMMA/5(Column_5(1B)) -> 16_to_1_Byte_Multiplexer4/15
  Char_EXCLAMATION_MARK/5(Column_5(1B)) -> 16_to_1_Byte_Multiplexer4/13
  Char_QUESTION_MARK/5(Column_5(1B)) -> 16_to_1_Byte_Multiplexer4/14
  Char_QUOTE/5(Column_5(1B)) -> 16_to_1_Byte_Multiplexer4/12
  Char_SHARP/5(Column_5(1B)) -> 16_to_1_Byte_Multiplexer4/11
  Char_PERCENT/5(Column_5(1B)) -> 16_to_1_Byte_Multiplexer4/10
  Char_LEFT_PARENTHESES/5(Column_5(1B)) -> 16_to_1_Byte_Multiplexer4/9
  Char_RIGHT_PARENTHESES/5(Column_5(1B)) -> 16_to_1_Byte_Multiplexer4/8
  Char_SPACE/5(Column_5(1B)) -> 16_to_1_Byte_Multiplexer4/7
  Char_CURSOR/5(Column_5(1B)) -> 16_to_1_Byte_Multiplexer4/6
  Char_RECTANGLE/5(Column_5(1B)) -> 16_to_1_Byte_Multiplexer4/5
  Char_ARROW_DOWN/6(Column_6(1B)) -> 16_to_1_Byte_Multiplexer5/20
  Char_ARROW_LEFT/6(Column_6(1B)) -> 16_to_1_Byte_Multiplexer5/19
  Char_ARROW_RIGHT/6(Column_6(1B)) -> 16_to_1_Byte_Multiplexer5/18
  Char_UNDERSCORE/6(Column_6(1B)) -> 16_to_1_Byte_Multiplexer5/17
  Char_DOT/6(Column_6(1B)) -> 16_to_1_Byte_Multiplexer5/16
  Char_COMMA/6(Column_6(1B)) -> 16_to_1_Byte_Multiplexer5/15
  Char_QUESTION_MARK/6(Column_6(1B)) -> 16_to_1_Byte_Multiplexer5/14
  Char_EXCLAMATION_MARK/6(Column_6(1B)) -> 16_to_1_Byte_Multiplexer5/13
  Char_QUOTE/6(Column_6(1B)) -> 16_to_1_Byte_Multiplexer5/12
  Char_SHARP/6(Column_6(1B)) -> 16_to_1_Byte_Multiplexer5/11
  Char_PERCENT/6(Column_6(1B)) -> 16_to_1_Byte_Multiplexer5/10
  Char_LEFT_PARENTHESES/6(Column_6(1B)) -> 16_to_1_Byte_Multiplexer5/9
  Char_RIGHT_PARENTHESES/7(Column_7(1B)) -> 16_to_1_Byte_Multiplexer6/8
  Char_RIGHT_PARENTHESES/6(Column_6(1B)) -> 16_to_1_Byte_Multiplexer5/8
  Char_SPACE/6(Column_6(1B)) -> 16_to_1_Byte_Multiplexer5/7
  Char_CURSOR/6(Column_6(1B)) -> 16_to_1_Byte_Multiplexer5/6
  Char_RECTANGLE/6(Column_6(1B)) -> 16_to_1_Byte_Multiplexer5/5
  Char_ARROW_DOWN/7(Column_7(1B)) -> 16_to_1_Byte_Multiplexer6/20
  Char_ARROW_LEFT/7(Column_7(1B)) -> 16_to_1_Byte_Multiplexer6/19
  Char_ARROW_RIGHT/7(Column_7(1B)) -> 16_to_1_Byte_Multiplexer6/18
  Char_UNDERSCORE/7(Column_7(1B)) -> 16_to_1_Byte_Multiplexer6/17
  Char_DOT/7(Column_7(1B)) -> 16_to_1_Byte_Multiplexer6/16
  Char_COMMA/7(Column_7(1B)) -> 16_to_1_Byte_Multiplexer6/15
  Char_QUESTION_MARK/7(Column_7(1B)) -> 16_to_1_Byte_Multiplexer6/14
  Char_EXCLAMATION_MARK/7(Column_7(1B)) -> 16_to_1_Byte_Multiplexer6/13
  Char_QUOTE/7(Column_7(1B)) -> 16_to_1_Byte_Multiplexer6/12
  Char_SHARP/7(Column_7(1B)) -> 16_to_1_Byte_Multiplexer6/11
  Char_PERCENT/7(Column_7(1B)) -> 16_to_1_Byte_Multiplexer6/10
  Char_LEFT_PARENTHESES/7(Column_7(1B)) -> 16_to_1_Byte_Multiplexer6/9
  Char_SPACE/7(Column_7(1B)) -> 16_to_1_Byte_Multiplexer6/7
  Char_CURSOR/7(Column_7(1B)) -> 16_to_1_Byte_Multiplexer6/6
  Char_RECTANGLE/7(Column_7(1B)) -> 16_to_1_Byte_Multiplexer6/5
  Char_ARROW_DOWN/8(Column_8(1B)) -> 16_to_1_Byte_Multiplexer7/20
  Char_ARROW_LEFT/8(Column_8(1B)) -> 16_to_1_Byte_Multiplexer7/19
  Char_ARROW_RIGHT/8(Column_8(1B)) -> 16_to_1_Byte_Multiplexer7/18
  Char_UNDERSCORE/8(Column_8(1B)) -> 16_to_1_Byte_Multiplexer7/17
  Char_DOT/8(Column_8(1B)) -> 16_to_1_Byte_Multiplexer7/16
  Char_COMMA/8(Column_8(1B)) -> 16_to_1_Byte_Multiplexer7/15
  Char_QUESTION_MARK/8(Column_8(1B)) -> 16_to_1_Byte_Multiplexer7/14
  Char_EXCLAMATION_MARK/8(Column_8(1B)) -> 16_to_1_Byte_Multiplexer7/13
  Char_QUOTE/8(Column_8(1B)) -> 16_to_1_Byte_Multiplexer7/12
  Char_SHARP/8(Column_8(1B)) -> 16_to_1_Byte_Multiplexer7/11
  Char_PERCENT/8(Column_8(1B)) -> 16_to_1_Byte_Multiplexer7/10
  Char_LEFT_PARENTHESES/8(Column_8(1B)) -> 16_to_1_Byte_Multiplexer7/9
  Char_RIGHT_PARENTHESES/8(Column_8(1B)) -> 16_to_1_Byte_Multiplexer7/8
  Char_SPACE/8(Column_8(1B)) -> 16_to_1_Byte_Multiplexer7/7
  Char_CURSOR/8(Column_8(1B)) -> 16_to_1_Byte_Multiplexer7/6
  Char_RECTANGLE/8(Column_8(1B)) -> 16_to_1_Byte_Multiplexer7/5
  16_to_1_Byte_Multiplexer/1 -> Column_1(1B)/1
  16_to_1_Byte_Multiplexer1/1 -> Column_2(1B)/1
  16_to_1_Byte_Multiplexer2/1 -> Column_3(1B)/1
  16_to_1_Byte_Multiplexer3/1 -> Column_4(1B)/1
  16_to_1_Byte_Multiplexer4/1 -> Column_5(1B)/1
  16_to_1_Byte_Multiplexer5/1 -> Column_6(1B)/1
  16_to_1_Byte_Multiplexer6/1 -> Column_7(1B)/1
  16_to_1_Byte_Multiplexer7/1 -> Column_8(1B)/1
  Address_0_In(1b)/1 -> 16_to_1_Byte_Multiplexer/4, 16_to_1_Byte_Multiplexer1/4, 16_to_1_Byte_Multiplexer2/4, 16_to_1_Byte_Multiplexer3/4, 16_to_1_Byte_Multiplexer4/4, 16_to_1_Byte_Multiplexer5/4, 16_to_1_Byte_Multiplexer6/4, 16_to_1_Byte_Multiplexer7/4
  Address_1_In(1b)/1 -> 16_to_1_Byte_Multiplexer/3, 16_to_1_Byte_Multiplexer1/3, 16_to_1_Byte_Multiplexer2/3, 16_to_1_Byte_Multiplexer3/3, 16_to_1_Byte_Multiplexer4/3, 16_to_1_Byte_Multiplexer5/3, 16_to_1_Byte_Multiplexer6/3, 16_to_1_Byte_Multiplexer7/3
  Address_2_In(1b)/1 -> 16_to_1_Byte_Multiplexer/2, 16_to_1_Byte_Multiplexer1/2, 16_to_1_Byte_Multiplexer2/2, 16_to_1_Byte_Multiplexer3/2, 16_to_1_Byte_Multiplexer4/2, 16_to_1_Byte_Multiplexer5/2, 16_to_1_Byte_Multiplexer6/2, 16_to_1_Byte_Multiplexer7/2
  Address_3_In(1b)/1 -> 16_to_1_Byte_Multiplexer/1, 16_to_1_Byte_Multiplexer1/1, 16_to_1_Byte_Multiplexer2/1, 16_to_1_Byte_Multiplexer3/1, 16_to_1_Byte_Multiplexer4/1, 16_to_1_Byte_Multiplexer5/1, 16_to_1_Byte_Multiplexer6/1, 16_to_1_Byte_Multiplexer7/1

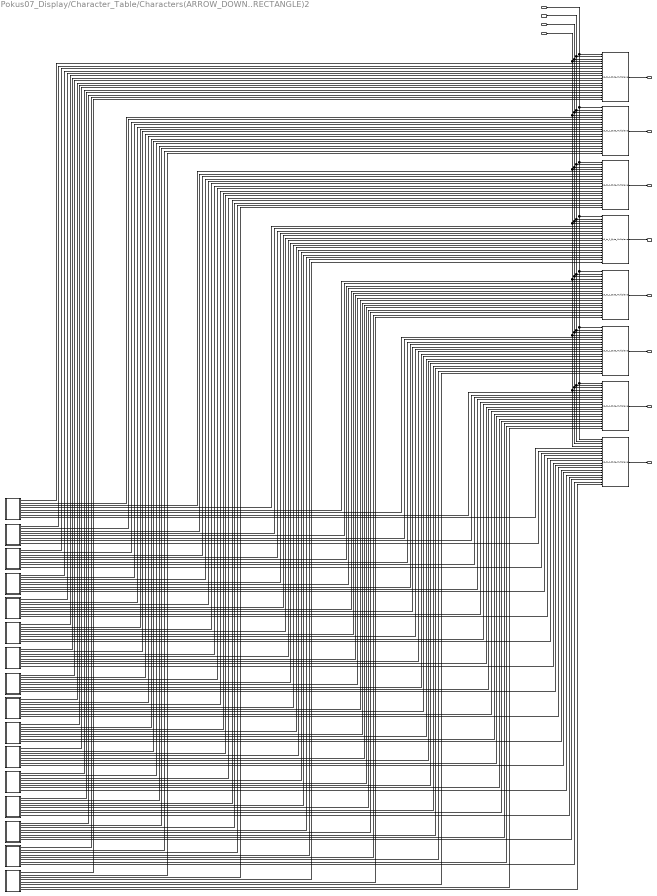
== system Pokus07_Display/Character_Table/Characters(ARROW_DOWN..RECTANGLE)2 ==
  Address_3_In(1b) : Inport
  Address_2_In(1b) : Inport  Port=2
  Address_1_In(1b) : Inport  Port=3
  Address_0_In(1b) : Inport  Port=4
  16_to_1_Byte_Multiplexer{,1..7} (8 alike) : Common_Library/Multiplexers/16_to_1_Byte_Multiplexer
  Char_ARROW_DOWN : Subsystem
  Char_ARROW_LEFT : Subsystem
  Char_ARROW_RIGHT : Subsystem
  Char_COMMA : Subsystem
  Char_CURSOR : Subsystem
  Char_DOT : Subsystem
  Char_EXCLAMATION_MARK : Subsystem
  Char_LEFT_PARENTHESES : Subsystem
  Char_PERCENT : Subsystem
  Char_QUESTION_MARK : Subsystem
  Char_QUOTE : Subsystem
  Char_RECTANGLE : Subsystem
  Char_RIGHT_PARENTHESES : Subsystem
  Char_SHARP : Subsystem
  Char_SPACE : Subsystem
  Char_UNDERSCORE : Subsystem
  Column_1(1B) : Outport
  Column_2(1B) : Outport  Port=2
  Column_3(1B) : Outport  Port=3
  Column_4(1B) : Outport  Port=4
  Column_5(1B) : Outport  Port=5
  Column_6(1B) : Outport  Port=6
  Column_7(1B) : Outport  Port=7
  Column_8(1B) : Outport  Port=8
  wires:
  Char_RECTANGLE/1(Column_1(1B)) -> 16_to_1_Byte_Multiplexer/5
  Char_CURSOR/1(Column_1(1B)) -> 16_to_1_Byte_Multiplexer/6
  Char_SPACE/1(Column_1(1B)) -> 16_to_1_Byte_Multiplexer/7
  Char_RIGHT_PARENTHESES/1(Column_1(1B)) -> 16_to_1_Byte_Multiplexer/8
  Char_LEFT_PARENTHESES/1(Column_1(1B)) -> 16_to_1_Byte_Multiplexer/9
  Char_PERCENT/1(Column_1(1B)) -> 16_to_1_Byte_Multiplexer/10
  Char_SHARP/1(Column_1(1B)) -> 16_to_1_Byte_Multiplexer/11
  Char_QUOTE/1(Column_1(1B)) -> 16_to_1_Byte_Multiplexer/12
  Char_EXCLAMATION_MARK/1(Column_1(1B)) -> 16_to_1_Byte_Multiplexer/13
  Char_QUESTION_MARK/1(Column_1(1B)) -> 16_to_1_Byte_Multiplexer/14
  Char_COMMA/1(Column_1(1B)) -> 16_to_1_Byte_Multiplexer/15
  Char_DOT/1(Column_1(1B)) -> 16_to_1_Byte_Multiplexer/16
  Char_UNDERSCORE/1(Column_1(1B)) -> 16_to_1_Byte_Multiplexer/17
  Char_ARROW_RIGHT/1(Column_1(1B)) -> 16_to_1_Byte_Multiplexer/18
  Char_ARROW_LEFT/1(Column_1(1B)) -> 16_to_1_Byte_Multiplexer/19
  Char_ARROW_DOWN/1(Column_1(1B)) -> 16_to_1_Byte_Multiplexer/20
  Char_RECTANGLE/2(Column_2(1B)) -> 16_to_1_Byte_Multiplexer1/5
  Char_ARROW_DOWN/2(Column_2(1B)) -> 16_to_1_Byte_Multiplexer1/20
  Char_ARROW_LEFT/2(Column_2(1B)) -> 16_to_1_Byte_Multiplexer1/19
  Char_ARROW_RIGHT/2(Column_2(1B)) -> 16_to_1_Byte_Multiplexer1/18
  Char_UNDERSCORE/2(Column_2(1B)) -> 16_to_1_Byte_Multiplexer1/17
  Char_DOT/2(Column_2(1B)) -> 16_to_1_Byte_Multiplexer1/16
  Char_COMMA/2(Column_2(1B)) -> 16_to_1_Byte_Multiplexer1/15
  Char_QUESTION_MARK/2(Column_2(1B)) -> 16_to_1_Byte_Multiplexer1/14
  Char_EXCLAMATION_MARK/2(Column_2(1B)) -> 16_to_1_Byte_Multiplexer1/13
  Char_QUOTE/2(Column_2(1B)) -> 16_to_1_Byte_Multiplexer1/12
  Char_SHARP/2(Column_2(1B)) -> 16_to_1_Byte_Multiplexer1/11
  Char_PERCENT/2(Column_2(1B)) -> 16_to_1_Byte_Multiplexer1/10
  Char_LEFT_PARENTHESES/2(Column_2(1B)) -> 16_to_1_Byte_Multiplexer1/9
  Char_RIGHT_PARENTHESES/2(Column_2(1B)) -> 16_to_1_Byte_Multiplexer1/8
  Char_SPACE/2(Column_2(1B)) -> 16_to_1_Byte_Multiplexer1/7
  Char_CURSOR/2(Column_2(1B)) -> 16_to_1_Byte_Multiplexer1/6
  Char_ARROW_DOWN/3(Column_3(1B)) -> 16_to_1_Byte_Multiplexer2/20
  Char_ARROW_LEFT/3(Column_3(1B)) -> 16_to_1_Byte_Multiplexer2/19
  Char_ARROW_RIGHT/3(Column_3(1B)) -> 16_to_1_Byte_Multiplexer2/18
  Char_UNDERSCORE/3(Column_3(1B)) -> 16_to_1_Byte_Multiplexer2/17
  Char_DOT/3(Column_3(1B)) -> 16_to_1_Byte_Multiplexer2/16
  Char_COMMA/3(Column_3(1B)) -> 16_to_1_Byte_Multiplexer2/15
  Char_QUESTION_MARK/3(Column_3(1B)) -> 16_to_1_Byte_Multiplexer2/14
  Char_EXCLAMATION_MARK/3(Column_3(1B)) -> 16_to_1_Byte_Multiplexer2/13
  Char_QUOTE/3(Column_3(1B)) -> 16_to_1_Byte_Multiplexer2/12
  Char_SHARP/3(Column_3(1B)) -> 16_to_1_Byte_Multiplexer2/11
  Char_PERCENT/3(Column_3(1B)) -> 16_to_1_Byte_Multiplexer2/10
  Char_LEFT_PARENTHESES/3(Column_3(1B)) -> 16_to_1_Byte_Multiplexer2/9
  Char_RIGHT_PARENTHESES/3(Column_3(1B)) -> 16_to_1_Byte_Multiplexer2/8
  Char_SPACE/3(Column_3(1B)) -> 16_to_1_Byte_Multiplexer2/7
  Char_CURSOR/3(Column_3(1B)) -> 16_to_1_Byte_Multiplexer2/6
  Char_RECTANGLE/3(Column_3(1B)) -> 16_to_1_Byte_Multiplexer2/5
  Char_ARROW_DOWN/4(Column_4(1B)) -> 16_to_1_Byte_Multiplexer3/20
  Char_ARROW_LEFT/4(Column_4(1B)) -> 16_to_1_Byte_Multiplexer3/19
  Char_ARROW_RIGHT/4(Column_4(1B)) -> 16_to_1_Byte_Multiplexer3/18
  Char_UNDERSCORE/4(Column_4(1B)) -> 16_to_1_Byte_Multiplexer3/17
  Char_DOT/4(Column_4(1B)) -> 16_to_1_Byte_Multiplexer3/16
  Char_COMMA/4(Column_4(1B)) -> 16_to_1_Byte_Multiplexer3/15
  Char_QUESTION_MARK/4(Column_4(1B)) -> 16_to_1_Byte_Multiplexer3/14
  Char_EXCLAMATION_MARK/4(Column_4(1B)) -> 16_to_1_Byte_Multiplexer3/13
  Char_QUOTE/4(Column_4(1B)) -> 16_to_1_Byte_Multiplexer3/12
  Char_SHARP/4(Column_4(1B)) -> 16_to_1_Byte_Multiplexer3/11
  Char_PERCENT/4(Column_4(1B)) -> 16_to_1_Byte_Multiplexer3/10
  Char_LEFT_PARENTHESES/4(Column_4(1B)) -> 16_to_1_Byte_Multiplexer3/9
  Char_RIGHT_PARENTHESES/4(Column_4(1B)) -> 16_to_1_Byte_Multiplexer3/8
  Char_SPACE/4(Column_4(1B)) -> 16_to_1_Byte_Multiplexer3/7
  Char_CURSOR/4(Column_4(1B)) -> 16_to_1_Byte_Multiplexer3/6
  Char_RECTANGLE/4(Column_4(1B)) -> 16_to_1_Byte_Multiplexer3/5
  Char_ARROW_DOWN/5(Column_5(1B)) -> 16_to_1_Byte_Multiplexer4/20
  Char_ARROW_LEFT/5(Column_5(1B)) -> 16_to_1_Byte_Multiplexer4/19
  Char_ARROW_RIGHT/5(Column_5(1B)) -> 16_to_1_Byte_Multiplexer4/18
  Char_UNDERSCORE/5(Column_5(1B)) -> 16_to_1_Byte_Multiplexer4/17
  Char_DOT/5(Column_5(1B)) -> 16_to_1_Byte_Multiplexer4/16
  Char_COMMA/5(Column_5(1B)) -> 16_to_1_Byte_Multiplexer4/15
  Char_EXCLAMATION_MARK/5(Column_5(1B)) -> 16_to_1_Byte_Multiplexer4/13
  Char_QUESTION_MARK/5(Column_5(1B)) -> 16_to_1_Byte_Multiplexer4/14
  Char_QUOTE/5(Column_5(1B)) -> 16_to_1_Byte_Multiplexer4/12
  Char_SHARP/5(Column_5(1B)) -> 16_to_1_Byte_Multiplexer4/11
  Char_PERCENT/5(Column_5(1B)) -> 16_to_1_Byte_Multiplexer4/10
  Char_LEFT_PARENTHESES/5(Column_5(1B)) -> 16_to_1_Byte_Multiplexer4/9
  Char_RIGHT_PARENTHESES/5(Column_5(1B)) -> 16_to_1_Byte_Multiplexer4/8
  Char_SPACE/5(Column_5(1B)) -> 16_to_1_Byte_Multiplexer4/7
  Char_CURSOR/5(Column_5(1B)) -> 16_to_1_Byte_Multiplexer4/6
  Char_RECTANGLE/5(Column_5(1B)) -> 16_to_1_Byte_Multiplexer4/5
  Char_ARROW_DOWN/6(Column_6(1B)) -> 16_to_1_Byte_Multiplexer5/20
  Char_ARROW_LEFT/6(Column_6(1B)) -> 16_to_1_Byte_Multiplexer5/19
  Char_ARROW_RIGHT/6(Column_6(1B)) -> 16_to_1_Byte_Multiplexer5/18
  Char_UNDERSCORE/6(Column_6(1B)) -> 16_to_1_Byte_Multiplexer5/17
  Char_DOT/6(Column_6(1B)) -> 16_to_1_Byte_Multiplexer5/16
  Char_COMMA/6(Column_6(1B)) -> 16_to_1_Byte_Multiplexer5/15
  Char_QUESTION_MARK/6(Column_6(1B)) -> 16_to_1_Byte_Multiplexer5/14
  Char_EXCLAMATION_MARK/6(Column_6(1B)) -> 16_to_1_Byte_Multiplexer5/13
  Char_QUOTE/6(Column_6(1B)) -> 16_to_1_Byte_Multiplexer5/12
  Char_SHARP/6(Column_6(1B)) -> 16_to_1_Byte_Multiplexer5/11
  Char_PERCENT/6(Column_6(1B)) -> 16_to_1_Byte_Multiplexer5/10
  Char_LEFT_PARENTHESES/6(Column_6(1B)) -> 16_to_1_Byte_Multiplexer5/9
  Char_RIGHT_PARENTHESES/7(Column_7(1B)) -> 16_to_1_Byte_Multiplexer6/8
  Char_RIGHT_PARENTHESES/6(Column_6(1B)) -> 16_to_1_Byte_Multiplexer5/8
  Char_SPACE/6(Column_6(1B)) -> 16_to_1_Byte_Multiplexer5/7
  Char_CURSOR/6(Column_6(1B)) -> 16_to_1_Byte_Multiplexer5/6
  Char_RECTANGLE/6(Column_6(1B)) -> 16_to_1_Byte_Multiplexer5/5
  Char_ARROW_DOWN/7(Column_7(1B)) -> 16_to_1_Byte_Multiplexer6/20
  Char_ARROW_LEFT/7(Column_7(1B)) -> 16_to_1_Byte_Multiplexer6/19
  Char_ARROW_RIGHT/7(Column_7(1B)) -> 16_to_1_Byte_Multiplexer6/18
  Char_UNDERSCORE/7(Column_7(1B)) -> 16_to_1_Byte_Multiplexer6/17
  Char_DOT/7(Column_7(1B)) -> 16_to_1_Byte_Multiplexer6/16
  Char_COMMA/7(Column_7(1B)) -> 16_to_1_Byte_Multiplexer6/15
  Char_QUESTION_MARK/7(Column_7(1B)) -> 16_to_1_Byte_Multiplexer6/14
  Char_EXCLAMATION_MARK/7(Column_7(1B)) -> 16_to_1_Byte_Multiplexer6/13
  Char_QUOTE/7(Column_7(1B)) -> 16_to_1_Byte_Multiplexer6/12
  Char_SHARP/7(Column_7(1B)) -> 16_to_1_Byte_Multiplexer6/11
  Char_PERCENT/7(Column_7(1B)) -> 16_to_1_Byte_Multiplexer6/10
  Char_LEFT_PARENTHESES/7(Column_7(1B)) -> 16_to_1_Byte_Multiplexer6/9
  Char_SPACE/7(Column_7(1B)) -> 16_to_1_Byte_Multiplexer6/7
  Char_CURSOR/7(Column_7(1B)) -> 16_to_1_Byte_Multiplexer6/6
  Char_RECTANGLE/7(Column_7(1B)) -> 16_to_1_Byte_Multiplexer6/5
  Char_ARROW_DOWN/8(Column_8(1B)) -> 16_to_1_Byte_Multiplexer7/20
  Char_ARROW_LEFT/8(Column_8(1B)) -> 16_to_1_Byte_Multiplexer7/19
  Char_ARROW_RIGHT/8(Column_8(1B)) -> 16_to_1_Byte_Multiplexer7/18
  Char_UNDERSCORE/8(Column_8(1B)) -> 16_to_1_Byte_Multiplexer7/17
  Char_DOT/8(Column_8(1B)) -> 16_to_1_Byte_Multiplexer7/16
  Char_COMMA/8(Column_8(1B)) -> 16_to_1_Byte_Multiplexer7/15
  Char_QUESTION_MARK/8(Column_8(1B)) -> 16_to_1_Byte_Multiplexer7/14
  Char_EXCLAMATION_MARK/8(Column_8(1B)) -> 16_to_1_Byte_Multiplexer7/13
  Char_QUOTE/8(Column_8(1B)) -> 16_to_1_Byte_Multiplexer7/12
  Char_SHARP/8(Column_8(1B)) -> 16_to_1_Byte_Multiplexer7/11
  Char_PERCENT/8(Column_8(1B)) -> 16_to_1_Byte_Multiplexer7/10
  Char_LEFT_PARENTHESES/8(Column_8(1B)) -> 16_to_1_Byte_Multiplexer7/9
  Char_RIGHT_PARENTHESES/8(Column_8(1B)) -> 16_to_1_Byte_Multiplexer7/8
  Char_SPACE/8(Column_8(1B)) -> 16_to_1_Byte_Multiplexer7/7
  Char_CURSOR/8(Column_8(1B)) -> 16_to_1_Byte_Multiplexer7/6
  Char_RECTANGLE/8(Column_8(1B)) -> 16_to_1_Byte_Multiplexer7/5
  16_to_1_Byte_Multiplexer/1 -> Column_1(1B)/1
  16_to_1_Byte_Multiplexer1/1 -> Column_2(1B)/1
  16_to_1_Byte_Multiplexer2/1 -> Column_3(1B)/1
  16_to_1_Byte_Multiplexer3/1 -> Column_4(1B)/1
  16_to_1_Byte_Multiplexer4/1 -> Column_5(1B)/1
  16_to_1_Byte_Multiplexer5/1 -> Column_6(1B)/1
  16_to_1_Byte_Multiplexer6/1 -> Column_7(1B)/1
  16_to_1_Byte_Multiplexer7/1 -> Column_8(1B)/1
  Address_0_In(1b)/1 -> 16_to_1_Byte_Multiplexer/4, 16_to_1_Byte_Multiplexer1/4, 16_to_1_Byte_Multiplexer2/4, 16_to_1_Byte_Multiplexer3/4, 16_to_1_Byte_Multiplexer4/4, 16_to_1_Byte_Multiplexer5/4, 16_to_1_Byte_Multiplexer6/4, 16_to_1_Byte_Multiplexer7/4
  Address_1_In(1b)/1 -> 16_to_1_Byte_Multiplexer/3, 16_to_1_Byte_Multiplexer1/3, 16_to_1_Byte_Multiplexer2/3, 16_to_1_Byte_Multiplexer3/3, 16_to_1_Byte_Multiplexer4/3, 16_to_1_Byte_Multiplexer5/3, 16_to_1_Byte_Multiplexer6/3, 16_to_1_Byte_Multiplexer7/3
  Address_2_In(1b)/1 -> 16_to_1_Byte_Multiplexer/2, 16_to_1_Byte_Multiplexer1/2, 16_to_1_Byte_Multiplexer2/2, 16_to_1_Byte_Multiplexer3/2, 16_to_1_Byte_Multiplexer4/2, 16_to_1_Byte_Multiplexer5/2, 16_to_1_Byte_Multiplexer6/2, 16_to_1_Byte_Multiplexer7/2
  Address_3_In(1b)/1 -> 16_to_1_Byte_Multiplexer/1, 16_to_1_Byte_Multiplexer1/1, 16_to_1_Byte_Multiplexer2/1, 16_to_1_Byte_Multiplexer3/1, 16_to_1_Byte_Multiplexer4/1, 16_to_1_Byte_Multiplexer5/1, 16_to_1_Byte_Multiplexer6/1, 16_to_1_Byte_Multiplexer7/1
